simulink library "Susp_AxleTA2PR"  (R2025b)
settings: Solver=VariableStepAuto  StartTime=0.0  StopTime=10.0  RelTol=1e-3
undefined symbols (not defined in the file): Init, Vehicle
libraries: Susp_AxleTA2PR_Linkage x1, sm_lib x1, Steer_DragLink x1
Description:
  | Component of Simscape Vehicle Templates Library
  | 
  | Copyright 2018-2025 The MathWorks, Inc.
settings Model: Creator=mwalker  LastModifiedBy=smiller
settings SolverCC: AlgebraicLoopSolver=TrustRegion
settings DataIOCC: ReturnWorkspaceOutputs=off
settings DebuggingCC: UnconnectedInputMsg=warning  UnconnectedOutputMsg=warning  UnconnectedLineMsg=warning  ArithmeticOperatorsInVariantConditions=warning
settings ModelReferenceCC: EnableRefExpFcnMdlSchedulingChecks=on
settings SFSimCC: CustomCodeUndefinedFunction=UseInterfaceOnly
settings RTWCC: GPUComputeCapability=3.5

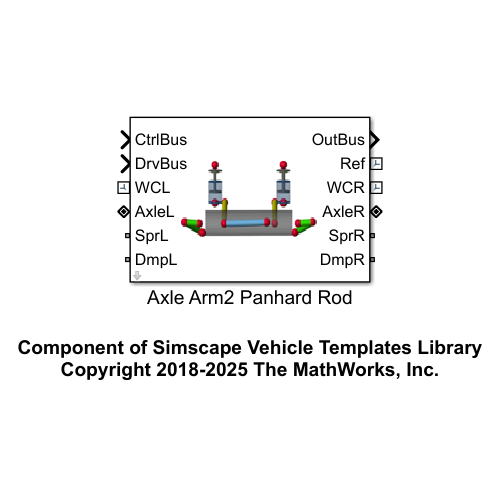
[thumbnail: Simulink's stored preview of the top-level diagram]
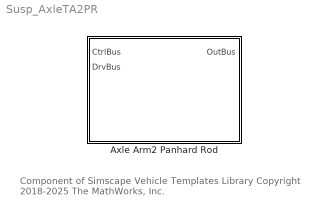
== system Susp_AxleTA2PR ==
  note: Component of Simscape Vehicle Templates Library
      | Copyright 2018-2025 The MathWorks, Inc.
  Axle Arm2 Panhard Rod : Subsystem  mask(Rigid Axle, Two Trailing Arms, Panhard Rod, with Steering System){Init=Init, Susp=Vehicle.Chassis.SuspA1}
      mask prompts: Init "Initial Values (structure)"; Susp "Susp (structure)"
      mask help: Models a rigid axle connected to the chassis with two trailing arms and a panhard rod, along with a steering system. The displacement of the springs and dampers are modeled here and the forces are modeled in a separate subsystem.
      mask Display: image('sm_car_vehicle_susp_axleta2pr_IMAGE.png');

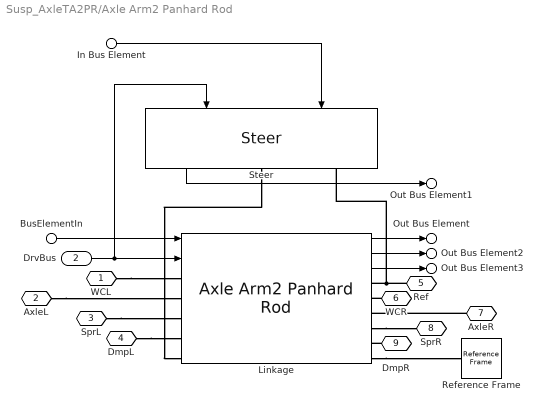
== system Susp_AxleTA2PR/Axle Arm2 Panhard Rod ==
  BusElementIn : Inport  PortName=CtrlBus
  In Bus Element : Inport  PortName=CtrlBus  Element=Steer
  DrvBus : Inport  Port=2
  Linkage : Susp_AxleTA2PR_Linkage/Axle Arm2 Panhard Rod  VariantControl=LiveAxle  Init=Init  hp_shock_top=Susp.AxleTA2PR.Shock.sTop.Value  hp_shock_bot=Susp.AxleTA2PR.Shock.sBottom.Value  hp_arm_body=Susp.AxleTA2PR.TrailingArm.sBody.Value  hp_arm_axle=Susp.AxleTA2PR.TrailingArm.sAxle.Value  hp_pan_body=Susp.AxleTA2PR.PanhardRod.sBody.Value  hp_pan_axle=Susp.AxleTA2PR.PanhardRod.sAxle.Value  hp_upr_axle=Susp.AxleTA2PR.Upright.sAxle.Value  hp_steerlink_out=Susp.AxleTA2PR.SteeringLink.sOutboard.Value  hp_axle_cg=Susp.AxleTA2PR.Axle.sCG.Value  hp_whl_ctr=Susp.AxleTA2PR.Upright.sWheelCentre.Value  hp_upr_drag=Susp.AxleTA2PR.Upright.sDragLink.Value  hp_chassis_bumpstop=Susp.AxleTA2PR.Bumpstop.sChassis.Value  hp_axle_bumpstop=Susp.AxleTA2PR.Bumpstop.sAxle.Value  aCaster=Susp.AxleTA2PR.Upright.aCaster.Value  aKPI=Susp.AxleTA2PR.Upright.aKPI.Value  axle_mass=Susp.AxleTA2PR.Axle.m.Value  arm_mass=Susp.AxleTA2PR.TrailingArm.m.Value  upr_mass=Susp.AxleTA2PR.Upright.m.Value  steerlink_mass=Susp.AxleTA2PR.SteeringLink.m.Value  panhard_mass=Susp.AxleTA2PR.PanhardRod.m.Value  Arm_to_Axle=Susp.AxleTA2PR.Arm_to_Axle  clr_arm=Visual.UpperArm.clr  opc_arm=Visual.part.opc  radius_arm=Visual.UpperArm.rad  clr_steerlink=Visual.SteeringRack.clr  opc_steerlink=Visual.part.opc  radius_steerlink=Visual.TrackRod.rad  clr_rod=Visual.Pushrod.clr  opc_rod=Visual.part.opc  radius_rod=Visual.Pushrod.rad  clr_conn_links=Visual.hp.clr  opc_conn_links=Visual.hp.opc  size_conn_links=Visual.hp.rad  clr_upr=Visual.Upright.clr  opc_upr=Visual.part.opc  radius_upr=Visual.Upright.rad  piston_mass=Susp.AxleTA2PR.Shock.mPiston.Value  cyl_mass=Susp.AxleTA2PR.Shock.mCylinder.Value  shock_xmax=Susp.AxleTA2PR.Endstop.xMax.Value  shock_xmin=Susp.AxleTA2PR.Endstop.xMin.Value  Shock_Connection=Susp.AxleTA2PR.Shock_Connection  Bumpstop_Type=Susp.AxleTA2PR.Bumpstop.class.Value  bumpstop_height=Susp.AxleTA2PR.Bumpstop.xHeight.Value  bumpstop_k=Susp.AxleTA2PR.Bumpstop.K.Value  bumpstop_d=Susp.AxleTA2PR.Bumpstop.d.Value  bumpstop_xTrans=Susp.AxleTA2PR.Bumpstop.xTransition.Value  bumpstop_ptcld=Susp.AxleTA2PR.Bumpstop.sPointCloud.Value
  Reference Frame : sm_lib/Frames and Transforms/Reference Frame
  Steer : Steer_DragLink/Steer  VariantControl=Steer  LabelModeActiveChoice=DragCrossWheelDriven  Steer=Susp.Steer  VariantLabel=Susp.Steer.class.Value
      settings: AttributesFormatString=%<ActiveVariant>
  WCL : PMIOPort  Side=Left
  AxleL : PMIOPort  Port=2  Side=Left
  SprL : PMIOPort  Port=3  Side=Left
  DmpL : PMIOPort  Port=4  Side=Left
  Ref : PMIOPort  Port=5  Side=Right
  WCR : PMIOPort  Port=6  Side=Right
  AxleR : PMIOPort  Port=7  Side=Right
  SprR : PMIOPort  Port=8  Side=Right
  DmpR : PMIOPort  Port=9  Side=Right
  Out Bus Element : Outport  PortName=OutBus  Element=Linkage
  Out Bus Element1 : Outport  PortName=OutBus  Element=Steer
  Out Bus Element2 : Outport  PortName=OutBus  Element=WhlL
  Out Bus Element3 : Outport  PortName=OutBus  Element=WhlR
  wires:
  BusElementIn/1 -> Linkage/1
  Steer/1 -> Out Bus Element1/1
  DrvBus/1 -> Steer/1, Linkage/2
  Linkage/1 -> Out Bus Element/1
  In Bus Element/1 -> Steer/2
  Linkage/2 -> Out Bus Element2/1
  Linkage/3 -> Out Bus Element3/1
  connections:
  Linkage/RConn4 -- SprR/RConn1
  WCR/RConn1 -- Linkage/RConn2
  AxleL/RConn1 -- Linkage/LConn2
  Linkage/RConn6 -- Reference Frame/RConn1
  Ref/RConn1 -- Steer/RConn2 -- Linkage/RConn1
  Steer/RConn1 -- Linkage/LConn5
  DmpL/RConn1 -- Linkage/LConn4
  WCL/RConn1 -- Linkage/LConn1
  AxleR/RConn1 -- Linkage/RConn3
  SprL/RConn1 -- Linkage/LConn3
  DmpR/RConn1 -- Linkage/RConn5
